simulink model "penduum"  (R2019b)
settings: Solver=VariableStepAuto  StartTime=0.0  StopTime=10.0  RelTol=1e-3
values from neighbouring files (symbols this model uses):
  Ac = [(A-B*K)]    [State_Space.m]
  Bc = [B]    [State_Space.m]
  K = lqr(A,B,Q,R)    [LQG.m]    (also in State_Space.m; frequency_domain.m = 35; root_locus_method.m = 20; rscale.m = k)
  Nbar = rscale(sys_ss,K)    [State_Space.m]    (also in rscale.m = Nu + K*Nx)
settings Model: Creator=Khojasteh Mirza  LastModifiedBy=Khojasteh Mirza

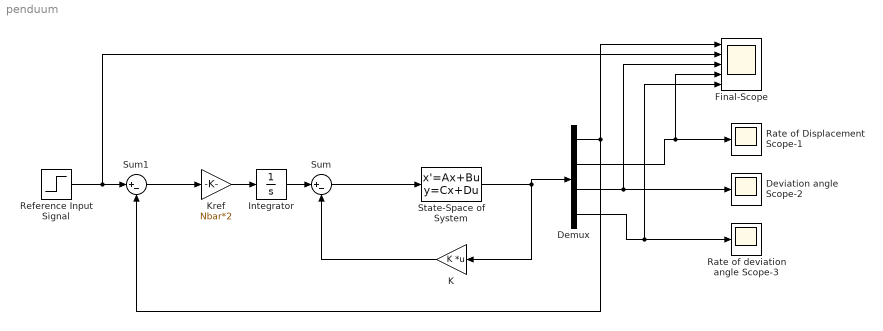
== system penduum ==
  Demux : Demux
  Deviation angle Scope-2 : Scope
  Final-Scope : Scope  NumInputPorts=5
  Integrator : Integrator
  K : Gain  Gain=K  Multiplication=Matrix(K*u)
  Kref : Gain  Gain=Nbar*2
  Rate of Displacement Scope-1 : Scope
  Rate of deviation angle Scope-3 : Scope
  Reference Input Signal : Step  After=0.5  SampleTime=0
  "State-Space of System " : StateSpace  A=Ac  B=Bc  C=eye(4)  D=[0;0;0;0]  InitialCondition=0
  Sum : Sum  Inputs=|+-
  Sum1 : Sum  Inputs=|+-
  wires:
  "State-Space of System "/1 -> Demux/1, K/1
  K/1 -> Sum/2
  Kref/1 -> Integrator/1
  Demux/1 -> Final-Scope/1, Sum1/2
  Demux/2 -> Final-Scope/4, Rate of Displacement Scope-1/1
  Demux/4 -> Rate of deviation angle Scope-3/1, Final-Scope/5
  Demux/3 -> Final-Scope/3, Deviation angle Scope-2/1
  Sum1/1 -> Kref/1
  Sum/1 -> "State-Space of System "/1
  Integrator/1 -> Sum/1
  Reference Input Signal/1 -> Final-Scope/2, Sum1/1
